simulink model "model2"  (R2020b)
settings: Solver=VariableStepAuto  StartTime=0.0  StopTime=20  MaxStep=1e-5  MinStep=1e-6  RelTol=1e-3
undefined symbols (not defined in the file or in its folder): i
settings Model: Creator=MSI  LastModifiedBy=MSI
settings SolverCC: InitialStep=1e-6

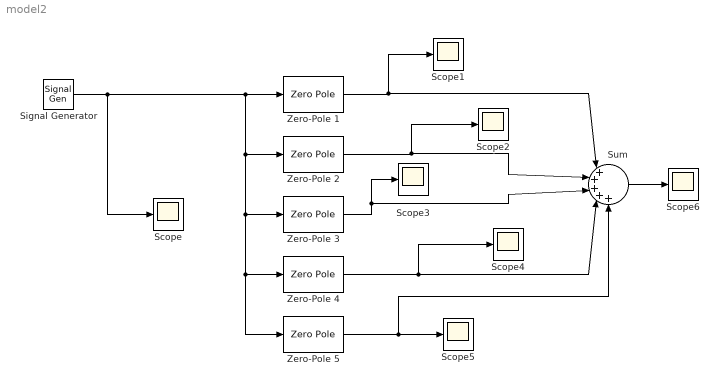
== system model2 ==
  Scope{,1..6} (7 alike) : Scope
  Signal Generator : SignalGenerator  WaveForm=square  Frequency=3
  Sum : Sum  Inputs=|+++++
  Zero-Pole 1 : ZeroPole  Zeros=[0]  Poles=[-1 * 2*pi*3*0.005+i*1*2*pi*3*0.9999875, -1*2*pi*3*0.005-i*1*2*pi*3*0.9999875]  Gain=[1*2*pi*3*0.01]
  Zero-Pole 2 : ZeroPole  Zeros=[0]  Poles=[-2 * 2*pi*3*0.005+i*2*2*pi*3*0.9999875, -2*2*pi*3*0.005-i*2*2*pi*3*0.9999875]  Gain=[2*2*pi*3*0.01]
  Zero-Pole 3 : ZeroPole  Zeros=[0]  Poles=[-3 * 2*pi*3*0.005+i*3*2*pi*3*0.9999875, -3*2*pi*3*0.005-i*3*2*pi*3*0.9999875]  Gain=[3*2*pi*3*0.01]
  Zero-Pole 4 : ZeroPole  Zeros=[0]  Poles=[-4 * 2*pi*3*0.005+i*4*2*pi*3*0.9999875, -4*2*pi*3*0.005-i*4*2*pi*3*0.9999875]  Gain=[4*2*pi*3*0.01]
  Zero-Pole 5 : ZeroPole  Zeros=[0]  Poles=[-5 * 2*pi*3*0.005+i*5*2*pi*3*0.9999875, -5*2*pi*3*0.005-i*5*2*pi*3*0.9999875]  Gain=[5*2*pi*3*0.01]
  wires:
  Signal Generator/1 -> Scope/1, Zero-Pole 5/1, Zero-Pole 4/1, Zero-Pole 3/1, Zero-Pole 2/1, Zero-Pole 1/1
  Zero-Pole 5/1 -> Sum/5, Scope5/1
  Zero-Pole 4/1 -> Sum/4, Scope4/1
  Zero-Pole 3/1 -> Sum/3, Scope3/1
  Zero-Pole 2/1 -> Sum/2, Scope2/1
  Zero-Pole 1/1 -> Sum/1, Scope1/1
  Sum/1 -> Scope6/1
